simulink model "PM_fnc21_Xdchg_Detection_TestHarness_backup1"  (R2022a)
settings: Solver=VariableStepAuto  StartTime=0.0  StopTime=10.0  RelTol=1e-3
values from neighbouring files (symbols this model uses):
  rate_ms = 10    [PM_fnc1000_tc01_iter01_testsignal_builder.m]    (also in PM_fnc21_tc01_iter01_testsignal_builder.m; PM_fnc22_tc01_iter01_testsignal_builder.m)
settings Model: Creator=306427  LastModifiedBy=306427

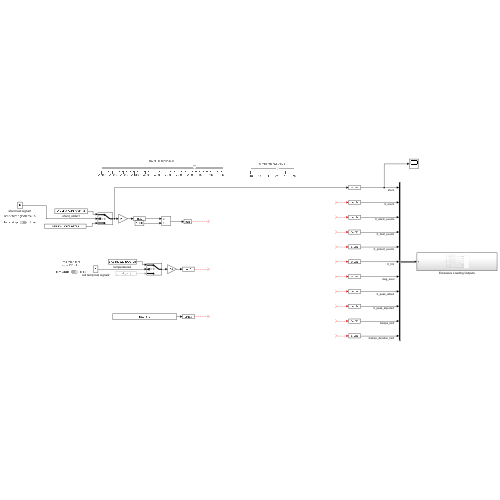
[thumbnail: Simulink's stored preview of the top-level diagram]
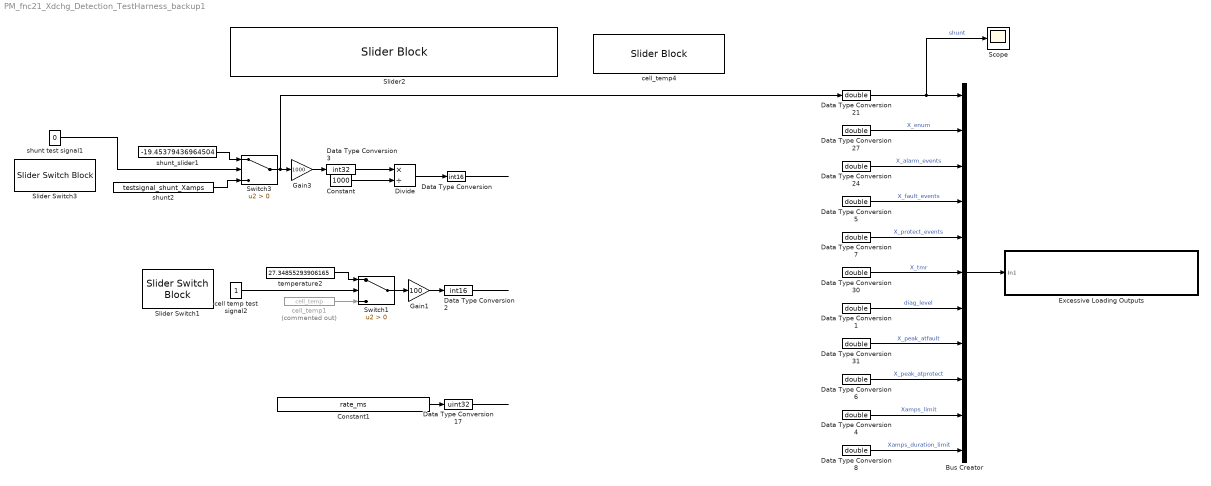
== system PM_fnc21_Xdchg_Detection_TestHarness_backup1 ==
  Bus Creator : BusCreator  Inputs=11
  Constant : Constant  Value=1000
  Constant1 : Constant  Value=rate_ms
  Data Type Conversion : DataTypeConversion  OutDataTypeStr=int16  SaturateOnIntegerOverflow=off  RndMeth=Floor
  Data Type Conversion{1,4..8,21,24,27,30..31} (11 alike) : DataTypeConversion  OutDataTypeStr=double  SaturateOnIntegerOverflow=off  RndMeth=Floor
  Data Type Conversion17 : DataTypeConversion  OutDataTypeStr=uint32  SaturateOnIntegerOverflow=off  RndMeth=Floor
  Data Type Conversion2 : DataTypeConversion  OutDataTypeStr=int16  SaturateOnIntegerOverflow=off  RndMeth=Floor
  Data Type Conversion3 : DataTypeConversion  OutDataTypeStr=int32  SaturateOnIntegerOverflow=off  RndMeth=Floor
  Divide : Product  Inputs=*/  OutDataTypeStr=int32  SaturateOnIntegerOverflow=on
  Excessive Loading Outputs : Subsystem
  Gain1 : Gain  Gain=100
  Gain3 : Gain  Gain=1000
  Scope : Scope
  Slider Switch1 : SliderSwitchBlock
      settings: Values={{'from wksp', 'slider'}, [0 1]}
  Slider Switch3 : SliderSwitchBlock
      settings: Values={{'from wksp', 'slider'}, [0 1]}
  Slider2 : SliderBlock  ScaleMin=-1700  ScaleMax=+500
  Switch1 : Switch  Criteria=u2 > Threshold  SaturateOnIntegerOverflow=off  InputSameDT=off
  Switch3 : Switch  Criteria=u2 > Threshold  SaturateOnIntegerOverflow=off  InputSameDT=off
  cell temp test signal2 : Constant
  cell_temp1 : FromWorkspace  Commented=on  VariableName=cell_temp  OutDataTypeStr=double  SampleTime=[0, 1]
  cell_temp4 : SliderBlock  ScaleMin=-40  ScaleMax=70
  shunt test signal1 : Constant  Value=0
  shunt2 : FromWorkspace  VariableName=testsignal_shunt_Xamps  OutDataTypeStr=double
  shunt_slider1 : Constant  Value=-19.45379436964504  OutDataTypeStr=double
  temperature2 : Constant  Value=27.34855293906165  OutDataTypeStr=double
  wires:
  ? -> Data Type Conversion4/1
  Data Type Conversion7/1 -> Bus Creator/5  "X_protect_events"
  Data Type Conversion1/1 -> Bus Creator/7  "diag_level"
  ? -> Data Type Conversion1/1
  ? -> Data Type Conversion7/1
  Data Type Conversion/1 -> ?
  cell_temp1/1 -> Switch1/3
  Divide/1 -> Data Type Conversion/1
  ? -> Data Type Conversion27/1
  shunt_slider1/1 -> Switch3/1
  ? -> Data Type Conversion8/1
  Data Type Conversion3/1 -> Divide/1
  Gain1/1 -> Data Type Conversion2/1
  Switch1/1 -> Gain1/1
  shunt2/1 -> Switch3/3
  ? -> Data Type Conversion30/1
  Switch3/1 -> Data Type Conversion21/1, Gain3/1
  ? -> Data Type Conversion24/1
  Data Type Conversion21/1 -> Scope/1, Bus Creator/1  "shunt"
  ? -> Data Type Conversion5/1
  Data Type Conversion30/1 -> Bus Creator/6  "X_tmr"
  Data Type Conversion17/1 -> ?
  Data Type Conversion31/1 -> Bus Creator/8  "X_peak_atfault"
  Gain3/1 -> Data Type Conversion3/1
  Bus Creator/1 -> Excessive Loading Outputs/1(In1)
  cell temp test signal2/1 -> Switch1/2
  Data Type Conversion6/1 -> Bus Creator/9  "X_peak_atprotect"
  Constant/1 -> Divide/2
  Data Type Conversion4/1 -> Bus Creator/10  "Xamps_limit"
  Data Type Conversion5/1 -> Bus Creator/4  "X_fault_events"
  ? -> Data Type Conversion31/1
  Data Type Conversion27/1 -> Bus Creator/2  "X_enum"
  Data Type Conversion2/1 -> ?
  Data Type Conversion8/1 -> Bus Creator/11  "Xamps_duration_limit"
  Constant1/1 -> Data Type Conversion17/1
  Data Type Conversion24/1 -> Bus Creator/3  "X_alarm_events"
  shunt test signal1/1 -> Switch3/2
  temperature2/1 -> Switch1/1
  ? -> Data Type Conversion6/1

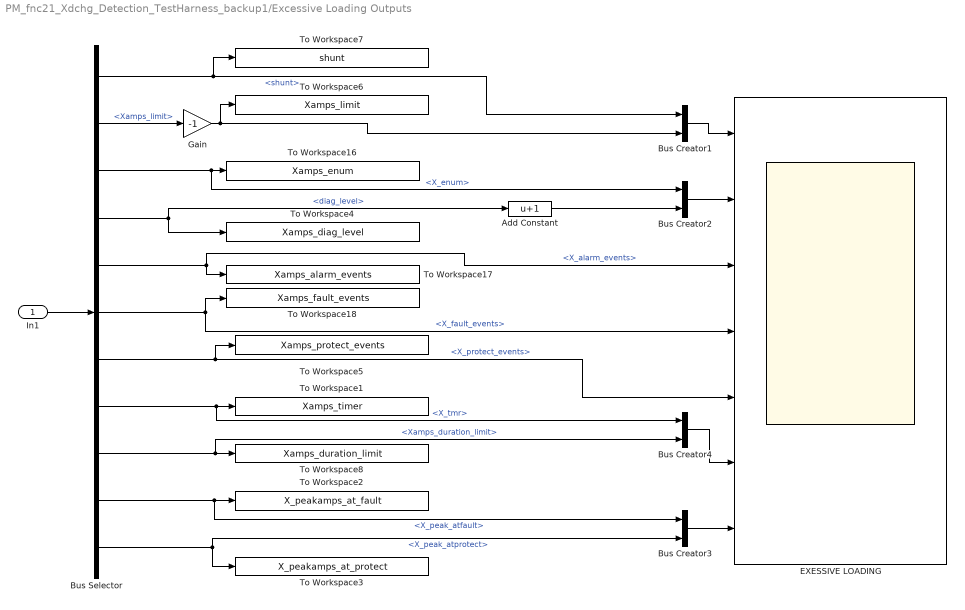
== system PM_fnc21_Xdchg_Detection_TestHarness_backup1/Excessive Loading Outputs ==
  In1 : Inport
  Add Constant : Bias  Bias=1  SaturateOnIntegerOverflow=off
  Bus Creator{1..4} (4 alike) : BusCreator  Inputs=2
  Bus Selector : BusSelector  OutputSignals=shunt,Xamps_limit,X_enum,diag_level,X_alarm_events,X_fault_events,X_protect_events,X_tmr,Xamps_duration_limit,X_peak_atfault,X_peak_atprotect
  EXESSIVE LOADING : Scope  NumInputPorts=7
  Gain : Gain  Gain=-1
  To Workspace1 : ToWorkspace  VariableName=Xamps_timer  SampleTime=-1
      settings: Save2DSignal=2-D array (concatenate along first dimension)
  To Workspace16 : ToWorkspace  VariableName=Xamps_enum  SampleTime=-1
      settings: Save2DSignal=2-D array (concatenate along first dimension)
  To Workspace17 : ToWorkspace  VariableName=Xamps_alarm_events  SampleTime=-1
      settings: Save2DSignal=2-D array (concatenate along first dimension)
  To Workspace18 : ToWorkspace  VariableName=Xamps_fault_events  SampleTime=-1
      settings: Save2DSignal=2-D array (concatenate along first dimension)
  To Workspace2 : ToWorkspace  VariableName=X_peakamps_at_fault  SampleTime=-1
      settings: Save2DSignal=2-D array (concatenate along first dimension)
  To Workspace3 : ToWorkspace  VariableName=X_peakamps_at_protect  SampleTime=-1
      settings: Save2DSignal=2-D array (concatenate along first dimension)
  To Workspace4 : ToWorkspace  VariableName=Xamps_diag_level  SampleTime=-1
      settings: Save2DSignal=2-D array (concatenate along first dimension)
  To Workspace5 : ToWorkspace  VariableName=Xamps_protect_events  SampleTime=-1
      settings: Save2DSignal=2-D array (concatenate along first dimension)
  To Workspace6 : ToWorkspace  VariableName=Xamps_limit  SampleTime=-1
      settings: Save2DSignal=2-D array (concatenate along first dimension)
  To Workspace7 : ToWorkspace  VariableName=shunt  SampleTime=-1
      settings: Save2DSignal=2-D array (concatenate along first dimension)
  To Workspace8 : ToWorkspace  VariableName=Xamps_duration_limit  SampleTime=-1
      settings: Save2DSignal=2-D array (concatenate along first dimension)
  wires:
  In1/1 -> Bus Selector/1
  Bus Selector/3 -> Bus Creator2/1, To Workspace16/1  "<X_enum>"
  Gain/1 -> To Workspace6/1, Bus Creator1/2
  Bus Selector/5 -> EXESSIVE LOADING/3, To Workspace17/1  "<X_alarm_events>"
  Bus Creator1/1 -> EXESSIVE LOADING/1
  Bus Selector/1 -> To Workspace7/1, Bus Creator1/1  "<shunt>"
  Bus Selector/6 -> To Workspace18/1, EXESSIVE LOADING/4  "<X_fault_events>"
  Bus Selector/8 -> Bus Creator4/1, To Workspace1/1  "<X_tmr>"
  Bus Selector/10 -> To Workspace2/1, Bus Creator3/1  "<X_peak_atfault>"
  Bus Selector/2 -> Gain/1  "<Xamps_limit>"
  Bus Selector/4 -> Add Constant/1, To Workspace4/1  "<diag_level>"
  Bus Selector/11 -> To Workspace3/1, Bus Creator3/2  "<X_peak_atprotect>"
  Bus Selector/7 -> To Workspace5/1, EXESSIVE LOADING/5  "<X_protect_events>"
  Bus Creator2/1 -> EXESSIVE LOADING/2
  Bus Creator3/1 -> EXESSIVE LOADING/7
  Add Constant/1 -> Bus Creator2/2
  Bus Selector/9 -> To Workspace8/1, Bus Creator4/2  "<Xamps_duration_limit>"
  Bus Creator4/1 -> EXESSIVE LOADING/6
